simulink model "Esys"  (R2016b)
settings: Solver=ode45  StartTime=0.0  StopTime=5  RelTol=1e-6  AbsTol=1e-6  EnableMultiTasking=on
values from neighbouring files (symbols this model uses):
  A = [A11,A12;A21,A22]    [Esys_Parameter.m]    (also in aufgabe1.m = double(subs(A)); aufgabe10.m = [-1 2; -2 -6]; aufgabe2.m = [0 1; -k/m -c/m]; aufgabe4.m = double(subs(subs(subs(A), [Uc1, Uc2], [Uc1r, Uc2r]))))
  bd = [0;1/(C2*R2)]    [Esys_Parameter.m]    (also in aufgabe1.m = double(subs(bd)); aufgabe4.m = double(subs(subs(subs(bd), [Uc1, Uc2], [Uc1r, Uc2r]))))
  bu = [1/(C1*R1);0]    [Esys_Parameter.m]    (also in aufgabe1.m = double(subs(bu)); aufgabe4.m = double(subs(subs(subs(bu), [Uc1, Uc2], [Uc1r, Uc2r]))))
  C1_ref = 1e-6    (= 1e-06)    [Esys_Parameter.m]    (also in Esys_S_m.m = block.DialogPrm(6).Data; aufgabe4.m)
  C2 = 1e-6    (= 1e-06)    [Esys_Parameter.m]    (also in Esys_S_m.m = block.DialogPrm(9).Data; aufgabe1.m; aufgabe4.m)
  K = 3    [Esys_Parameter.m]    (also in Esys_S_m.m = block.DialogPrm(5).Data; aufgabe1.m; aufgabe4.m)
  kC1 = 800e-9    (= 8e-07)    [Esys_Parameter.m]    (also in Esys_S_m.m = block.DialogPrm(8).Data; aufgabe4.m)
  R1 = 625    [Esys_Parameter.m]    (also in Esys_S_m.m = block.DialogPrm(3).Data; aufgabe1.m; aufgabe4.m)
  R2 = 3500    [Esys_Parameter.m]    (also in Esys_S_m.m = block.DialogPrm(4).Data; aufgabe1.m; aufgabe4.m)
  te = 1    [Esys_Parameter.m]
  ts = 3    [Esys_Parameter.m]
  UaR = K*UC2R    (= 15)    [Esys_Parameter.m]
  UC1_ref = -10    [Esys_Parameter.m]    (also in Esys_S_m.m = block.DialogPrm(7).Data; aufgabe4.m)
  UC1R = -(K*R2*UeR - R1*UsR - 2*R2*UeR + K*R1*UsR + K*R2*UsR)/(R1 + 2*R2)    (= -10)    [Esys_Parameter.m]
  UC2R = (R2*UeR + R1*UsR + R2*UsR)/(R1 + 2*R2)    (= 5)    [Esys_Parameter.m]
  Ue = 7    [Esys_Parameter.m]    (also in Esys_S_m.m = u(1))
  UeR = 5    [Esys_Parameter.m]    (also in aufgabe4.m)
  Us = 1    [Esys_Parameter.m]    (also in Esys_S_m.m = u(2))
  Usinus = 0.1    [Esys_Parameter.m]
  UsR = 5    [Esys_Parameter.m]    (also in aufgabe4.m)
  we = 10    [Esys_Parameter.m]
settings Model: Creator=sj  LastModifiedBy=M
settings DataIOCC: LimitDataPoints=on  SaveFormat=Array
settings OptimizationCC: LifeSpan=inf
settings DebuggingCC: SFUnexpectedBacktrackingDiag=warning  SFNoUnconditionalDefaultTransitionDiag=warning  SFExecutionAtInitializationDiag=none
settings HardwareCC: ProdBitPerPointer=32  ProdBitPerSizeT=32  ProdBitPerPtrDiffT=32  ProdLargestAtomicFloat=None  ProdIntDivRoundTo=Undefined  ProdEndianess=Unspecified  ProdWordSize=32  ProdHWDeviceType=32-bit Generic
settings ModelReferenceCC: PropagateSignalLabelsOutOfModel=off
settings GRTTargetCC: TargetLangStandard=C89/C90 (ANSI)  GeneratePreprocessorConditionals=Disable all
settings ConfigComp: CovMetricSettings=dw  CovHtmlReporting=on  CovSaveCumulativeToWorkspaceVar=on  CovSaveSingleToWorkspaceVar=on  CovExternalEMLEnable=off

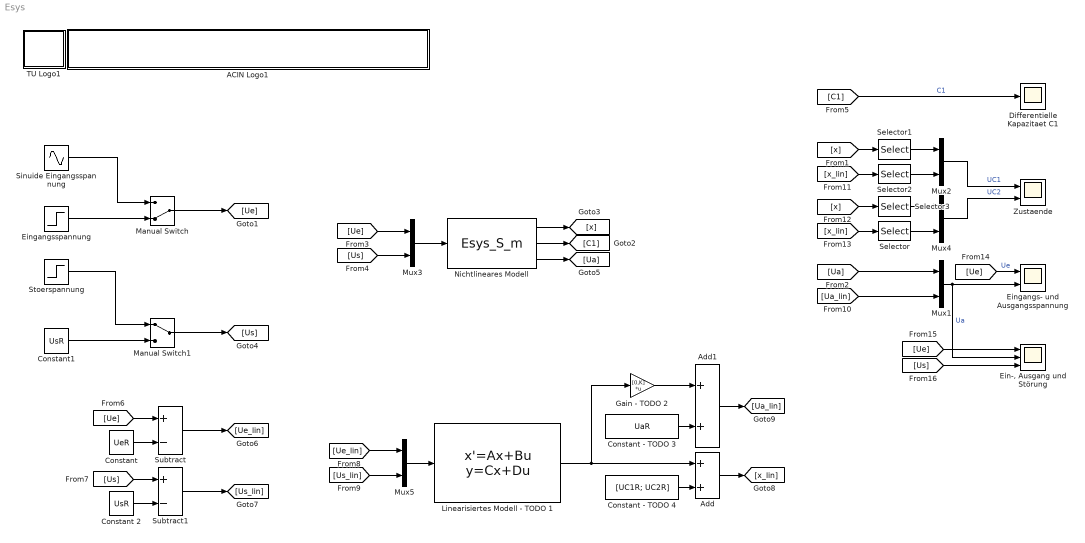
== system Esys ==
  ACIN Logo1 : Subsystem
      mask init:
      | s = get_param(gcb,'UserData');
      mask Display:
      | image(s.logo,[0 0 439 45]);
      | %axis image
  Add : Sum
  Add1 : Sum
  Constant : Constant  Value=UeR
  Constant - TODO 3 : Constant  Value=UaR
  Constant - TODO 4 : Constant  Value=[UC1R; UC2R]
  Constant 2 : Constant  Value=UsR
  Constant1 : Constant  Value=UsR
  Differentielle Kapazitaet C1 : Scope
  "Ein-, Ausgang und Störung" : Scope  NumInputPorts=3
  Eingangs- und Ausgangsspannung : Scope  NumInputPorts=2
  Eingangsspannung : Step  Time=te  Before=UeR  After=Ue  SampleTime=0
  Gain - TODO 2 : Gain  Gain=[0,K]  Multiplication=Matrix(K*u)
  Linearisiertes Modell - TODO 1 : StateSpace  A=A  B=[bu bd]  C=[1 0; 0 1]  D=[0 0; 0 0]  X0=[0;0]
  Manual Switch : ManualSwitch  CurrentSetting=0
  Manual Switch1 : ManualSwitch
  Mux{1..5} (5 alike) : Mux  Inputs=2
  Nichtlineares Modell : M-S-Function  FunctionName=Esys_S_m  Parameters=UC1R,UC2R,R1,R2,K,C1_ref,UC1_ref,kC1,C2  mask{UC10=UC1R, UC20=UC2R, R1=R1, R2=R2, K=K, C1_ref=C1_ref, UC1_ref=UC1_ref, kC1=kC1, C2=C2}
      mask prompts: UC10 "Anfangswert von UC1 in Volt"; UC20 "Anfangswert von UC2 in Volt"; R1 "Widerstand R1 in Ohm"; R2 "Widerstand R2 in Ohm"; K "Spannungsverstärkung K"; C1_ref "Kapazitäts-Referenzwert auf Kennlinie von C1 in F"; UC1_ref "Spannungs-Referenzwert auf Kennlinie von C1 in V"; kC1 "Steigung der Kennlinie in F/V"; C2 "Kapazität C2 in F"
      mask DialogControl Container3 Prompt: Nichtlineare Kapazität C1
  Selector : Selector  InputPortWidth=2  IndexOptions=Index vector (dialog)  Indices=2  OutputSizes=1
  Selector1 : Selector  InputPortWidth=2  IndexOptions=Index vector (dialog)  Indices=1  OutputSizes=1
  Selector2 : Selector  InputPortWidth=2  IndexOptions=Index vector (dialog)  Indices=1  OutputSizes=1
  Selector3 : Selector  InputPortWidth=2  IndexOptions=Index vector (dialog)  Indices=2  OutputSizes=1
  Sinuide Eingangsspannung : Sin  Amplitude=Usinus  Bias=UeR  Frequency=we  SampleTime=0
  Stoerspannung : Step  Time=ts  Before=UsR  After=Us  SampleTime=0
  Subtract : Sum  Inputs=+-
  Subtract1 : Sum  Inputs=+-
  TU Logo1 : Subsystem
      mask init:
      | s = get_param(gcb,'UserData');
      mask Display: image(s.logo,[0 0 45 45]);
  Zustaende : Scope  NumInputPorts=2
  wires:
  Mux3/1 -> Nichtlineares Modell/1
  Nichtlineares Modell/1 -> [x]
  Nichtlineares Modell/2 -> [C1]
  [Ue] -> Mux3/1
  [Us] -> Mux3/2
  Eingangsspannung/1 -> Manual Switch/2
  Sinuide Eingangsspannung/1 -> Manual Switch/1
  Manual Switch/1 -> [Ue]
  Nichtlineares Modell/3 -> [Ua]
  [C1] -> Differentielle Kapazitaet C1/1  "C1"
  Subtract/1 -> [Ue_lin]
  Constant/1 -> Subtract/2
  [Ue] -> Subtract/1
  Subtract1/1 -> [Us_lin]
  Constant 2/1 -> Subtract1/2
  [Us] -> Subtract1/1
  Linearisiertes Modell - TODO 1/1 -> Gain - TODO 2/1, Add/1
  Mux5/1 -> Linearisiertes Modell - TODO 1/1
  [Ue_lin] -> Mux5/1
  [Us_lin] -> Mux5/2
  Add/1 -> [x_lin]
  Constant - TODO 4/1 -> Add/2
  Gain - TODO 2/1 -> Add1/1
  Constant - TODO 3/1 -> Add1/2
  Add1/1 -> [Ua_lin]
  [Ua] -> Mux1/1
  [Ua_lin] -> Mux1/2
  Selector1/1 -> Mux2/1
  Selector2/1 -> Mux2/2
  [x] -> Selector1/1
  [x_lin] -> Selector2/1
  Selector3/1 -> Mux4/1
  Selector/1 -> Mux4/2
  [x] -> Selector3/1
  [x_lin] -> Selector/1
  Mux2/1 -> Zustaende/1  "UC1"
  Mux4/1 -> Zustaende/2  "UC2"
  [Ue] -> Eingangs- und Ausgangsspannung/1  "Ue"
  Mux1/1 -> "Ein-, Ausgang und Störung"/2, Eingangs- und Ausgangsspannung/2  "Ua"
  Manual Switch1/1 -> [Us]
  Stoerspannung/1 -> Manual Switch1/1
  Constant1/1 -> Manual Switch1/2
  [Ue] -> "Ein-, Ausgang und Störung"/1
  [Us] -> "Ein-, Ausgang und Störung"/3

== system Esys/ACIN Logo1 ==

== system Esys/TU Logo1 ==
